simulink library "lib_robot"  (R2022b)
settings: Solver=VariableStepAuto  StartTime=0.0  StopTime=10.0  RelTol=1e-3
values from neighbouring files (symbols this model uses):
  b = 5.8/6*1e-4    (= 9.66666666667e-05)    [DC_motor_mfile.m]
  J = 5.8e-7    (= 5.8e-07)    [DC_motor_mfile.m]
  K_D_pos = (2*zeta_m_pos*wn_m_pos*T - 1)/K    (= 0.0265230129141)    [DC_motor_mfile.m]
  K_I_cur = wn_m_cur^2 * T/K    (= 106000)    [DC_motor_mfile.m]
  K_I_pos = 0    [DC_motor_mfile.m]
  K_I_vel = wn_m_vel^2 * T/K    (= 39.4444444444)    [DC_motor_mfile.m]
  K_P_cur = (2*zeta_m_cur*wn_m_cur*T - 1)/K    (= 3.5)    [DC_motor_mfile.m]
  K_P_pos = wn_m_pos^2 * T/K    (= 9.86111111111)    [DC_motor_mfile.m]
  K_P_vel = (2*zeta_m_vel*wn_m_vel*T - 1)/K    (= 0.105411901803)    [DC_motor_mfile.m]
  Kb = 2.73e-3*(60/(2*pi))    (= 0.0260695796785)    [DC_motor_mfile.m]
  Km = 26.1e-3    (= 0.0261)    [DC_motor_mfile.m]
  La = 265e-6    (= 0.000265)    [DC_motor_mfile.m]
  Ra = 7.1    [DC_motor_mfile.m]
libraries: slpidlib x1
settings Model: Creator=chris  LastModifiedBy=chris

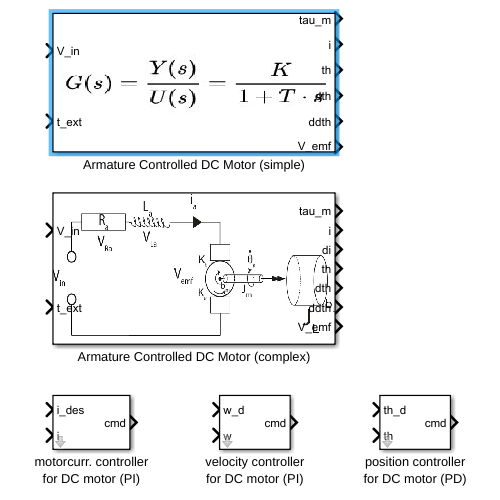
[thumbnail: Simulink's stored preview of the top-level diagram]
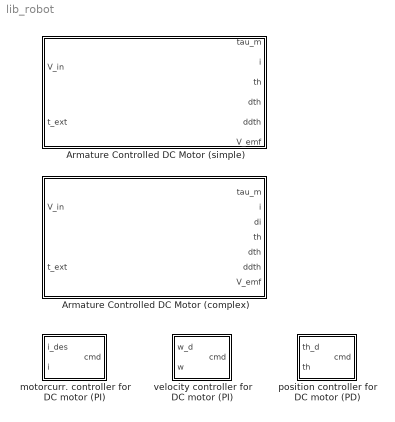
== system lib_robot ==
  Armature Controlled DC Motor (complex) : Subsystem
      mask Display: image('DC_motor_complex.png'); % Use "Edit Image" on toolstrip to change.
  Armature Controlled DC Motor (simple) : Subsystem
      mask Display: image('DC_motor_simple.jpg'); % Use "Edit Image" on toolstrip to change.
  motorcurr. controller for DC motor (PI) : Subsystem  mask{mask_K_P=K_P_cur, mask_K_I=K_I_cur}
      mask prompts: mask_K_P "value K_P"; mask_K_I "value K_I"
      mask TypeOptions mask_K_P: K_p/Gain
      mask TypeOptions mask_K_I: K_I/Gain
  position controller for DC motor (PD) : Subsystem  mask{P=K_P_pos, I=K_I_pos, D=K_D_pos, N=100}
      mask prompts: P "Simulink:masks:ProportionalP_MP"; I "Simulink:masks:IntegralI_MP"; D "Simulink:masks:DerivativeD_MP"; N "Simulink:masks:FilterCoefficientN_MP"
      mask TypeOptions P: PID Controller/P
      mask TypeOptions I: PID Controller/I
      mask TypeOptions D: PID Controller/D
      mask TypeOptions N: PID Controller/N
      mask DialogControl P Prompt: Proportional (P):
      mask DialogControl I Prompt: Integral (I):
      mask DialogControl D Prompt: Derivative (D):
      mask DialogControl N Prompt: Filter coefficient (N):
  velocity controller for DC motor (PI) : Subsystem  mask{mask_K_P=K_P_vel, mask_K_I=K_I_vel}
      mask prompts: mask_K_P "value K_P"; mask_K_I "vale K_I"
      mask TypeOptions mask_K_P: K_P/Gain
      mask TypeOptions mask_K_I: K_I/Gain

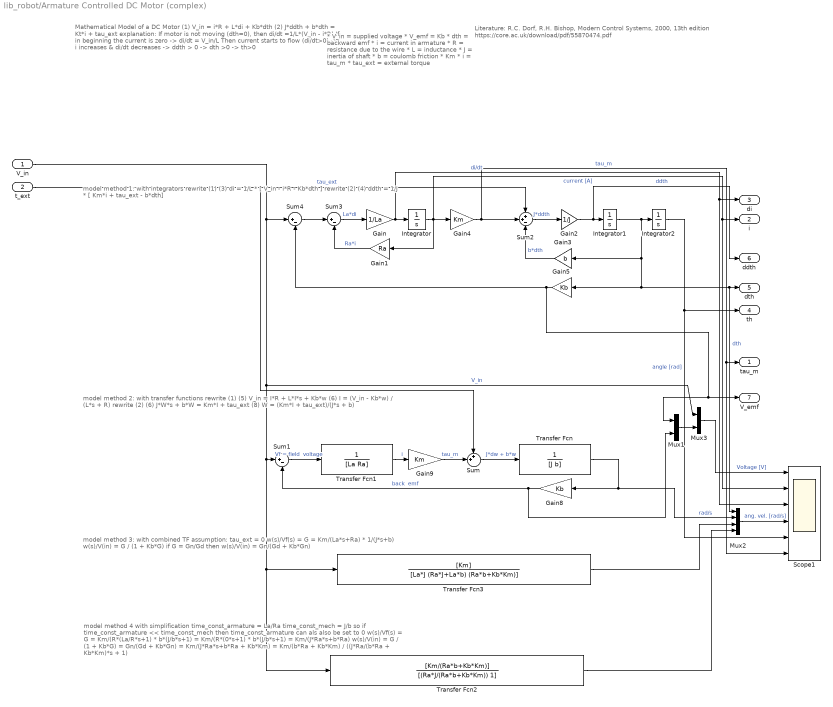
== system lib_robot/Armature Controlled DC Motor (complex) ==
  note: Mathematical Model of a DC Motor
      |
      | (1) V_in = i*R + L*di + Kb*dth
      | (2) J*ddth + b*dth = Kt*i + tau_ext
      |
      | explanation:
      |
      |  If motor is not moving (dth=0), then di/dt =1/L*(V_in - i*R)
      |  If in beginning the current is zero -> di/dt = V_in/L
      |
      |  Then current starts to flow (di/dt>0)
      |  -> i increases & di/dt decreases
      |  -> ddth > 0 -> dth >0 -> th>0
  note: model method 1: with integrators
      |
      | rewrite (1)
      | (3) di = 1/L * [ V_in - i*R - Kb*dth ]
      |
      | rewrite (2)
      | (4) ddth = 1/J * [ Km*i + tau_ext  - b*dth]
  note: model method 2: with transfer functions
      |
      | rewrite (1)
      |  (5) V_in = I*R + L*I*s + Kb*w
      |  (6) I = (V_in - Kb*w) / (L*s + R)
      |
      | rewrite (2)
      |  (6) J*W*s + b*W = Km*I + tau_ext
      |  (8) W = (Km*I + tau_ext)/(J*s + b)
  note: model method 3: with combined TF
      | assumption: tau_ext = 0
      |
      | w(s)/Vf(s) = G = Km/(La*s+Ra) * 1/(J*s+b)
      | w(s)/V(in) = G / (1 + Kb*G)
      |
      | if G = Gn/Gd
      | then w(s)/V(in) = Gn/(Gd + Kb*Gn)
  note: model method 4 with simplification
      |
      | time_const_armature = La/Ra
      | time_const_mech = J/b
      |
      | so if time_const_armature << time_const_mech
      | then time_const_armature can als also be set to 0
      |
      | w(s)/Vf(s) = G = Km/(R*(La/R*s+1) * b*(J/b*s+1)
      |                        = Km/(R*(0*s+1) * b*(J/b*s+1)
      |                        = Km/(J*Ra*s+b*Ra)
      |
      | w(s)/V(in) = G / (1 + Kb*G)
      |                 = Gn/(Gd + Kb*Gn)
      |                 = Km/(J*Ra*s+b*Ra + Kb*Km)
      |                 = Km/(b*Ra + Kb*Km) / ((J*Ra/(b*Ra + Kb*Km)*s + 1)
  note: * V_in = supplied voltage
      |  * V_emf = Kb * dth = backward emf
      |  * i = current in armature
      |  * R = resistance due to the wire
      |  * L = inductance
      |  * J = inertia of shaft
      |  * b = coulomb friction
      |  * Km * i = tau_m
      |  * tau_ext = external torque
  note: Literature:
      |
      | R.C. Dorf, R.H. Bishop, Modern Control Systems, 2000, 13th edition
      | https://core.ac.uk/download/pdf/55870474.pdf
  V_in : Inport
  t_ext : Inport  Port=2
  Gain : Gain  Gain=1/La
  Gain1 : Gain  Gain=Ra
  Gain2 : Gain  Gain=1/J
  Gain3 : Gain  Gain=b
  Gain4 : Gain  Gain=Km
  Gain5 : Gain  Gain=Kb
  Gain8 : Gain  Gain=Kb
  Gain9 : Gain  Gain=Km
  Integrator : Integrator
  Integrator1 : Integrator
  Integrator2 : Integrator
  Mux1 : Mux  Inputs=2
  Mux2 : Mux
  Mux3 : Mux  Inputs=2
  Scope1 : Scope  NumInputPorts=6
  Sum : Sum  Inputs=++|
  Sum1 : Sum  Inputs=|+-
  Sum2 : Sum  Inputs=++-
  Sum3 : Sum  Inputs=|+-
  Sum4 : Sum  Inputs=|+-
  Transfer Fcn : TransferFcn  Denominator=[J b]
  Transfer Fcn1 : TransferFcn  Denominator=[La Ra]
  Transfer Fcn2 : TransferFcn  Numerator=[Km/(Ra*b+Kb*Km)]  Denominator=[(Ra*J/(Ra*b+Kb*Km)) 1]
  Transfer Fcn3 : TransferFcn  Numerator=[Km]  Denominator=[La*J (Ra*J+La*b) (Ra*b+Kb*Km)]
  tau_m : Outport
  i : Outport  Port=2
  di : Outport  Port=3
  th : Outport  Port=4
  dth : Outport  Port=5
  ddth : Outport  Port=6
  V_emf : Outport  Port=7
  wires:
  Gain4/1 -> Sum2/2, Scope1/6, tau_m/1  "tau_m"
  Gain1/1 -> Sum3/2  "Ra*i"
  Gain3/1 -> Sum2/3  "b*dth"
  Gain2/1 -> ddth/1, Integrator1/1  "ddth"
  Gain/1 -> Integrator/1, di/1, Scope1/3  "di/dt"
  Integrator1/1 -> dth/1, Mux2/1, Gain5/1, Gain3/1, Integrator2/1  "dth"
  Sum3/1 -> Gain/1  "La*di"
  Sum2/1 -> Gain2/1  "J*ddth"
  Integrator2/1 -> th/1, Scope1/5  "angle [rad]"
  Gain5/1 -> Sum4/2, V_emf/1, Mux1/1
  Gain9/1 -> Sum/2  "tau_m"
  Sum/1 -> Transfer Fcn/1  "J*dw + b*w"
  Sum1/1 -> Transfer Fcn1/1  "Vf = field  voltage"
  Transfer Fcn1/1 -> Gain9/1  "i"
  Gain8/1 -> Sum1/2, Mux1/2  "back  emf"
  Transfer Fcn/1 -> Mux2/2, Gain8/1  "rad/s"
  V_in/1 -> Transfer Fcn2/1, Transfer Fcn3/1, Sum1/1, Mux3/1, Sum4/1  "V_in"
  t_ext/1 -> Sum2/1, Sum/1  "tau_ext"
  Integrator/1 -> Gain1/1, Gain4/1, i/1, Scope1/2  "current [A]"
  Mux2/1 -> Scope1/4  "ang. vel. [rad/s]"
  Mux3/1 -> Scope1/1  "Voltage [V]"
  Mux1/1 -> Mux3/2
  Transfer Fcn3/1 -> Mux2/3
  Transfer Fcn2/1 -> Mux2/4
  Sum4/1 -> Sum3/1

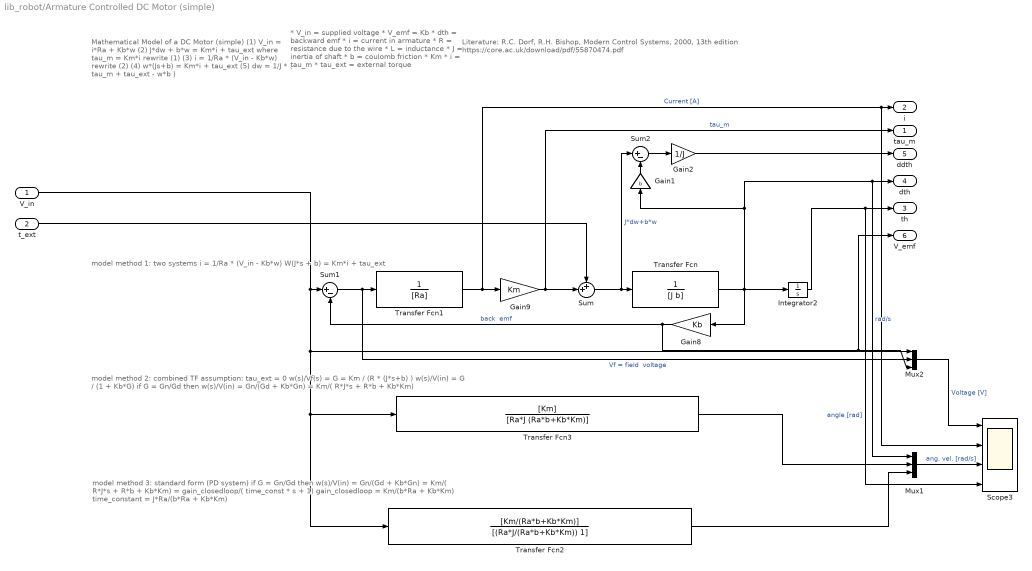
== system lib_robot/Armature Controlled DC Motor (simple) ==
  note: model method 3: standard form (PD system)
      |
      | if G = Gn/Gd
      | then w(s)/V(in) = Gn/(Gd + Kb*Gn)
      |  = Km/( R*J*s + R*b + Kb*Km)
      |  = gain_closedloop/( time_const * s + 1)
      |
      | gain_closedloop = Km/(b*Ra + Kb*Km)
      | time_constant     = J*Ra/(b*Ra + Kb*Km)
  note: model method 2: combined TF
      | assumption: tau_ext = 0
      |
      | w(s)/Vf(s) = G = Km / (R * (J*s+b) )
      | w(s)/V(in) = G / (1 + Kb*G)
      |
      | if G = Gn/Gd then w(s)/V(in) = Gn/(Gd + Kb*Gn)
      |  = Km/( R*J*s + R*b + Kb*Km)
  note: model method 1: two systems
      | i = 1/Ra * (V_in - Kb*w)
      | W(J*s + b)  = Km*i + tau_ext
  note: Mathematical Model of a DC Motor (simple)
      |
      | (1) V_in = i*Ra + Kb*w
      | (2) J*dw + b*w = Km*i + tau_ext
      | where tau_m = Km*i
      |
      | rewrite (1)
      | (3) i = 1/Ra * (V_in - Kb*w)
      |
      | rewrite (2)
      | (4) w*(Js+b) = Km*i + tau_ext
      | (5) dw = 1/J * ( tau_m + tau_ext - w*b )
  note: Literature:
      |
      | R.C. Dorf, R.H. Bishop, Modern Control Systems, 2000, 13th edition
      | https://core.ac.uk/download/pdf/55870474.pdf
  note: * V_in = supplied voltage
      |  * V_emf = Kb * dth = backward emf
      |  * i = current in armature
      |  * R = resistance due to the wire
      |  * L = inductance
      |  * J = inertia of shaft
      |  * b = coulomb friction
      |  * Km * i = tau_m
      |  * tau_ext = external torque
  V_in : Inport
  t_ext : Inport  Port=2
  Gain1 : Gain  Gain=b
  Gain2 : Gain  Gain=1/J
  Gain8 : Gain  Gain=Kb
  Gain9 : Gain  Gain=Km
  Integrator2 : Integrator
  Mux1 : Mux  Inputs=3
  Mux2 : Mux  Inputs=3
  Scope3 : Scope  NumInputPorts=4
  Sum : Sum  Inputs=++|
  Sum1 : Sum  Inputs=|+-
  Sum2 : Sum  Inputs=|+-
  Transfer Fcn : TransferFcn  Denominator=[J b]
  Transfer Fcn1 : TransferFcn  Denominator=[Ra]
  Transfer Fcn2 : TransferFcn  Numerator=[Km/(Ra*b+Kb*Km)]  Denominator=[(Ra*J/(Ra*b+Kb*Km)) 1]
  Transfer Fcn3 : TransferFcn  Numerator=[Km]  Denominator=[Ra*J (Ra*b+Kb*Km)]
  tau_m : Outport
  i : Outport  Port=2
  th : Outport  Port=3
  dth : Outport  Port=4
  ddth : Outport  Port=5
  V_emf : Outport  Port=6
  wires:
  Transfer Fcn2/1 -> Mux1/3
  Mux1/1 -> Scope3/3  "ang. vel. [rad/s]"
  Transfer Fcn3/1 -> Mux1/2
  t_ext/1 -> Sum/1
  V_in/1 -> Sum1/1, Transfer Fcn2/1, Transfer Fcn3/1, Mux2/1
  Transfer Fcn/1 -> Gain1/1, Mux1/1, dth/1, Integrator2/1, Gain8/1  "rad/s"
  Gain8/1 -> Sum1/2, V_emf/1, Mux2/3  "back  emf"
  Transfer Fcn1/1 -> Scope3/2, i/1, Gain9/1  "Current [A]"
  Sum1/1 -> Mux2/2, Transfer Fcn1/1  "Vf = field  voltage"
  Sum/1 -> Sum2/1, Transfer Fcn/1  "J*dw+b*w"
  Gain9/1 -> Sum/2, tau_m/1  "tau_m"
  Integrator2/1 -> Scope3/4, th/1  "angle [rad]"
  Sum2/1 -> Gain2/1
  Gain2/1 -> ddth/1
  Gain1/1 -> Sum2/2
  Mux2/1 -> Scope3/1  "Voltage [V]"

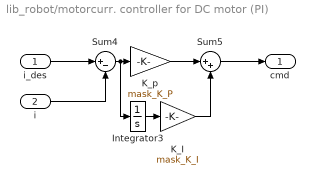
== system lib_robot/motorcurr. controller for DC motor (PI) ==
  i_des : Inport
  i : Inport  Port=2
  Integrator3 : Integrator
  K_I : Gain  Gain=mask_K_I
  K_p : Gain  Gain=mask_K_P
  Sum4 : Sum  Inputs=|+-
  Sum5 : Sum  Inputs=|++
  cmd : Outport
  wires:
  i_des/1 -> Sum4/1
  i/1 -> Sum4/2
  K_I/1 -> Sum5/2
  Integrator3/1 -> K_I/1
  Sum4/1 -> Integrator3/1, K_p/1
  K_p/1 -> Sum5/1
  Sum5/1 -> cmd/1

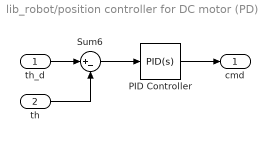
== system lib_robot/position controller for DC motor (PD) ==
  th_d : Inport
  th : Inport  Port=2
  PID Controller : slpidlib/PID Controller  Controller=PID  Form=Parallel  TimeDomain=Continuous-time  UseExternalTs=off  SampleTime=-1  IntegratorMethod=Forward Euler  FilterMethod=Forward Euler  ControllerParametersSource=internal  P=P  I=I  UseKiTs=off  D=D  N=N  UseFilter=on  TunerSelectOption=Transfer Function Based (PID Tuner App)  InitialConditionSource=internal  InitialConditionForIntegrator=0  InitialConditionForFilter=0  DifferentiatorICPrevScaledInput=0  ExternalReset=none  TrackingMode=off  Kt=1  LimitOutput=off  SatLimitsSource=internal  UpperSaturationLimit=inf  LowerSaturationLimit=-inf  LinearizeAsGain=on  AntiWindupMode=none  Kb=1  LimitIntegrator=off  UpperIntegratorSaturationLimit=inf  LowerIntegratorSaturationLimit=-inf  POutMin=[]  POutMax=[]  IOutMin=[]  IOutMax=[]  DOutMin=[]  DOutMax=[]  NOutMin=[]  NOutMax=[]  SumOutMin=[]  SumOutMax=[]  SaturationOutMin=[]  SaturationOutMax=[]  PParamMin=[]  PParamMax=[]  IParamMin=[]  IParamMax=[]  DParamMin=[]  DParamMax=[]  NParamMin=[]  NParamMax=[]  KbParamMin=[]  KbParamMax=[]  KtParamMin=[]  KtParamMax=[]  KbOutMin=[]  KbOutMax=[]  KtOutMin=[]  KtOutMax=[]  IntegratorOutMin=[]  IntegratorOutMax=[]  FilterOutMin=[]  FilterOutMax=[]  SumI1OutMin=[]  SumI1OutMax=[]  SumI2OutMin=[]  SumI2OutMax=[]  SumI3OutMin=[]  SumI3OutMax=[]  SumI4OutMin=[]  SumI4OutMax=[]  SumDOutMin=[]  SumDOutMax=[]  DifferentiatorOutMin=[]  DifferentiatorOutMax=[]  FilterDiffOutCoefMin=[]  FilterDiffOutCoefMax=[]  ReciprocalOutMin=[]  ReciprocalOutMax=[]  SumDenOutMin=[]  SumDenOutMax=[]  SumNumOutMin=[]  SumNumOutMax=[]  DivideOutMin=[]  DivideOutMax=[]  UdiffTsProdOutMin=[]  UdiffTsProdOutMax=[]  NTsProdOutMin=[]  NTsProdOutMax=[]  UintegralTsProdOutMin=[]  UintegralTsProdOutMax=[]  UngainTsProdOutMin=[]  UngainTsProdOutMax=[]  ClampingZeroOutDataTypeStr=Inherit: Inherit via back propagation  ClampingZeroOutMin=[]  ClampingZeroOutMax=[]  FilterDenConstantOutDataTypeStr=Inherit: Inherit via back propagation  FilterDenConstantOutMin=[]  FilterDenConstantOutMax=[]  PCopyOutDataTypeStr=Inherit: Inherit via back propagation  PCopyOutMin=[]  PCopyOutMax=[]  NCopyOutDataTypeStr=Inherit: Inherit via back propagation  NCopyOutMin=[]  NCopyOutMax=[]  IntegratorContinuousStateAttributes=''  IntegratorStateMustResolveToSignalObject=off  IntegratorRTWStateStorageClass=Auto  FilterContinuousStateAttributes=''  FilterStateMustResolveToSignalObject=off  FilterRTWStateStorageClass=Auto  ParallelPVariant=InternalParameters  IdealPVariant=Disabled  IVariant=InternalParameters  DVariant=InternalParameters  IntegratorVariant=Continuous  SatVariant=Disabled  AWVariant=Passthrough  PCopyVariant=Disabled  TRVariant=Disabled  FdbkBlocksVariant=Forward  IdealPFdbkVariant=Disabled  SatFdbkVariant=Disabled  DerivativeFilterVariant=ContFilter  NVariant=InternalParameters  NCopyVariant=Disabled  FilterICVariant=InternalICsFilter  IntegratorICVariant=InternalICs  ExternalResetVariant=Disabled  TRSumVariant=Passthrough  SumFdbkVariant=Disabled  SumVariant=Sum_PID  TsampFilterVariant=InternalTs  TsampNgainVariant=Passthrough  TsampIntegralVariant=Passthrough  ExternalSaturationOutDataTypeStr=Inherit: Same as second input
  Sum6 : Sum  Inputs=|+-
  cmd : Outport
  wires:
  PID Controller/1 -> cmd/1
  Sum6/1 -> PID Controller/1
  th/1 -> Sum6/2
  th_d/1 -> Sum6/1

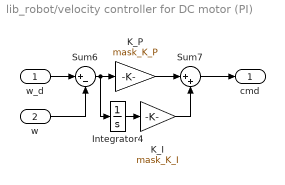
== system lib_robot/velocity controller for DC motor (PI) ==
  w_d : Inport
  w : Inport  Port=2
  Integrator4 : Integrator
  K_I : Gain  Gain=mask_K_I
  K_P : Gain  Gain=mask_K_P
  Sum6 : Sum  Inputs=|+-
  Sum7 : Sum  Inputs=|++
  cmd : Outport
  wires:
  Integrator4/1 -> K_I/1
  Sum7/1 -> cmd/1
  w/1 -> Sum6/2
  K_I/1 -> Sum7/2
  w_d/1 -> Sum6/1
  Sum6/1 -> K_P/1, Integrator4/1
  K_P/1 -> Sum7/1
